simulink model "TCLab_2018a"  (R2018a)
settings: Solver=FixedStepAuto  StartTime=0.0  StopTime=300  RelTol=1e-3  EnableMultiTasking=on
libraries: arduinolib x5
settings Model: EnablePacing=on  ExtModeTrigDuration=2  Creator=samvithr  LastModifiedBy=johnh
settings DataIOCC: ReturnWorkspaceOutputs=on
settings OptimizationCC: EnhancedBackFolding=on  PassReuseOutputArgsAs=Individual arguments  MaxStackSize=64  OptimizeBlockOrder=speed  DifferentSizesBufferReuse=on  OptimizationCustomize=off
settings DebuggingCC: ParameterTunabilityLossMsg=error
settings HardwareCC: ProdBitPerInt=16  ProdBitPerPointer=16  ProdBitPerSizeT=16  ProdBitPerPtrDiffT=16  ProdLargestAtomicFloat=None  ProdWordSize=8  ProdHWDeviceType=Atmel->AVR  UseEmbeddedCoderFeatures=off  UseSimulinkCoderFeatures=off
settings SFSimCC: SimUseLocalCustomCode=on  MATLABDynamicMemAlloc=off
settings RTWCC: SystemTargetFile=ert.tlc  HardwareBoard=Arduino Leonardo  TLCOptions=-aInlineSetEventsForThisBaseRateFcn=TLC_FALSE -aSuppressMultiTaskScheduler=TLC_FALSE -aRateBasedStepFcn=1  TemplateMakefile=ert_default_tmf  GenerateReport=on  RTWUseLocalCustomCode=on  Toolchain=Arduino AVR  BuildConfiguration=Faster Runs  IncludeHyperlinkInReport=on  LaunchReport=on  GenerateTraceInfo=on  GenerateTraceReport=on  GenerateTraceReportSl=on  GenerateTraceReportSf=on  GenerateTraceReportEml=on
settings CodeAppCC: ForceParamTrailComments=on  IgnoreCustomStorageClasses=off  OperatorAnnotations=on  SimulinkDataObjDesc=on  SFDataObjDesc=on  InsertBlockDesc=on
settings ERTTargetCC: SupportContinuousTime=on  SupportNonInlinedSFcns=on  SupportVariableSizeSignals=on  ExtModeStaticAllocSize=250

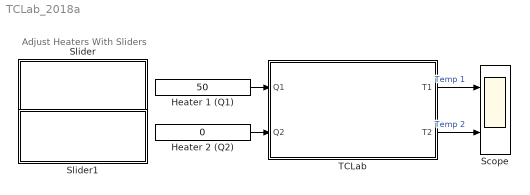
== system TCLab_2018a ==
  note: Adjust Heaters With Sliders
  Heater 1 (Q1) : Constant  Value=50
  Heater 2 (Q2) : Constant  Value=0
  Scope : Scope  NumInputPorts=2
  Slider : Subsystem  DialogController=hmiCreateDDGDialog  IsWebBlock=on  mask(MWDashboardBlock){webBlockId=4f456666-447b-466b-83de-2e1ef8be8358, webBlockType=slider, ShowInLibBrowser=on, ShowInitialText=on, HMISrcModelName=TCLab_2018a}
      mask prompts: webBlockId "WebBlock Id"; webBlockType "WebBlock Type"; HMISrcModelName "Source Model"
      mask help: Set value to tune parameters or variables.
      mask Help: helpview([docroot '/mapfiles/simulink.map'], 'hmi_slider')
      mask Display:
      | if strcmp(get_param(bdroot(gcb),'BlockDiagramType'),'library')
      |  image([(matlabroot) '/toolbox/simulink/hmi/icons/Slider.png'])
      | end
  Slider1 : Subsystem  DialogController=hmiCreateDDGDialog  IsWebBlock=on  mask(MWDashboardBlock){webBlockId=a74bbc03-d5d1-4ad2-8b84-f6283df9a75a, webBlockType=slider, ShowInLibBrowser=on, ShowInitialText=on, HMISrcModelName=TCLab_2018a}
      mask prompts: webBlockId "WebBlock Id"; webBlockType "WebBlock Type"; HMISrcModelName "Source Model"
      mask help: Set value to tune parameters or variables.
      mask Help: helpview([docroot '/mapfiles/simulink.map'], 'hmi_slider')
      mask Display:
      | if strcmp(get_param(bdroot(gcb),'BlockDiagramType'),'library')
      |  image([(matlabroot) '/toolbox/simulink/hmi/icons/Slider.png'])
      | end
  TCLab : Subsystem
      mask Display: image('Arduino.png');
  wires:
  Heater 2 (Q2)/1 -> TCLab/2(Q2)
  Heater 1 (Q1)/1 -> TCLab/1(Q1)
  TCLab/1(T1) -> Scope/1  "Temp 1"
  TCLab/2(T2) -> Scope/2  "Temp 2"

== system TCLab_2018a/Slider ==

== system TCLab_2018a/Slider1 ==

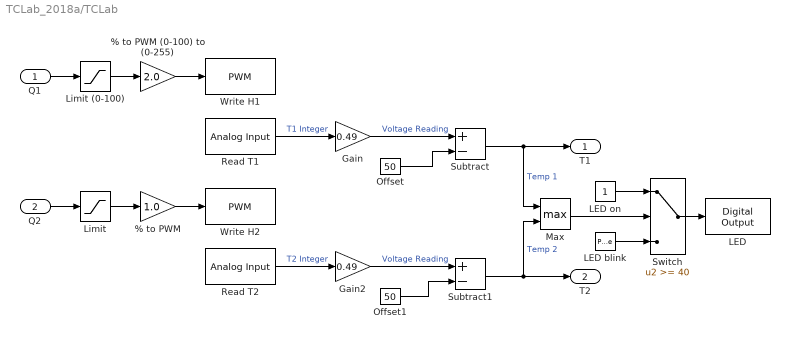
== system TCLab_2018a/TCLab ==
  Q1 : Inport
  Q2 : Inport  Port=2
  % to PWM (0-100) to (0-255) : Gain  Gain=2.0
  "% to PWM " : Gain  Gain=1.0
  Gain : Gain  Gain=0.49
  Gain2 : Gain  Gain=0.49
  LED : arduinolib/Digital Output  pinNumber=9  blockPlatform=arduino
  LED blink : DiscretePulseGenerator  Period=4  PulseWidth=2  SampleTime=0.5
  LED on : Constant
  Limit : Saturate  UpperLimit=100  LowerLimit=0
  Limit (0-100) : Saturate  UpperLimit=100  LowerLimit=0
  Max : MinMax  Function=max  Inputs=2
  Offset : Constant  Value=50
  Offset1 : Constant  Value=50
  Read T1 : arduinolib/Analog Input  pinNumber=0  ReadResultsOnly=off  ConversionTriggerSource=Software  ExternalTriggerType=uint32(0)  OutputDataType=uint16  EnableConversionCompleteNotify=off  EnableOuputStatus=off  SampleTime=0.5  blockPlatform=arduino
  Read T2 : arduinolib/Analog Input  pinNumber=2  ReadResultsOnly=off  ConversionTriggerSource=Software  ExternalTriggerType=uint32(0)  OutputDataType=uint16  EnableConversionCompleteNotify=off  EnableOuputStatus=off  SampleTime=0.5  blockPlatform=arduino
  Subtract : Sum  Inputs=+-
  Subtract1 : Sum  Inputs=+-
  Switch : Switch  Threshold=40
  Write H1 : arduinolib/PWM  pinNumber=3  EnableInputFrequency=off  InitialFrequency=2000  InitialDutyCycle=0  NotificationType=None  blockPlatform=arduino
  Write H2 : arduinolib/PWM  pinNumber=5  EnableInputFrequency=off  InitialFrequency=2000  InitialDutyCycle=0  NotificationType=None  blockPlatform=arduino
  T1 : Outport
  T2 : Outport  Port=2
  wires:
  Gain/1 -> Subtract/1  "Voltage Reading"
  Offset/1 -> Subtract/2
  Read T1/1 -> Gain/1  "T1 Integer"
  Subtract/1 -> Max/1, T1/1  "Temp 1"
  Limit (0-100)/1 -> % to PWM (0-100) to (0-255)/1
  % to PWM (0-100) to (0-255)/1 -> Write H1/1
  Switch/1 -> LED/1
  LED on/1 -> Switch/1
  LED blink/1 -> Switch/3
  Read T2/1 -> Gain2/1  "T2 Integer"
  Subtract1/1 -> Max/2, T2/1  "Temp 2"
  Gain2/1 -> Subtract1/1  "Voltage Reading"
  "% to PWM "/1 -> Write H2/1
  Offset1/1 -> Subtract1/2
  Max/1 -> Switch/2
  Q1/1 -> Limit (0-100)/1
  Q2/1 -> Limit/1
  Limit/1 -> "% to PWM "/1
